simulink model "BallAndPlate_RLSMPC_Controller"  (R2022b)
settings: configuration reference "controller_config_MPC" (kept outside this file)
undefined symbols (not defined in the file): BallAndPlate_ss_d, TimeStep_MPC, V_refNum
libraries: mpclib x1, sharedTrackingLibrary x1
settings Model: DataDictionary=BallAndPlate_system_data.sldd  Creator=tshintai  LastModifiedBy=tshintai
settings ConfigSetRef: SourceName=controller_config_MPC

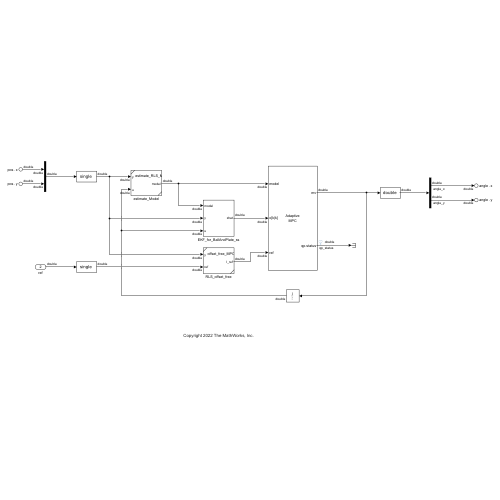
[thumbnail: Simulink's stored preview of the top-level diagram]
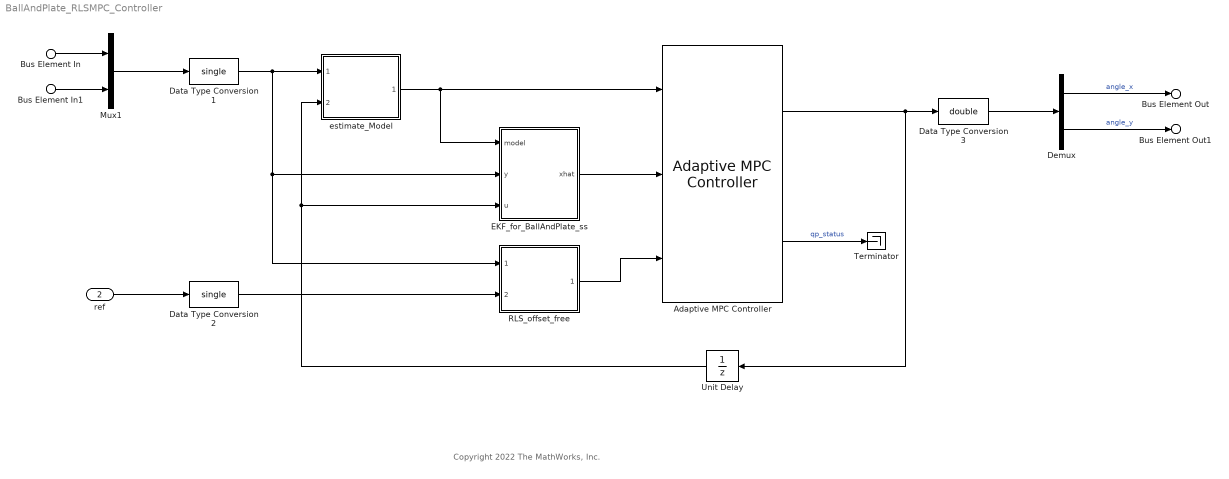
== system BallAndPlate_RLSMPC_Controller ==
  note: Copyright 2022 The MathWorks, Inc.
  Bus Element In : Inport  PortName=pos  Element=x
  Bus Element In1 : Inport  PortName=pos  Element=y
  ref : Inport  Port=2  OutDataTypeStr=double  PortDimensions=[2, V_refNum]
  Adaptive MPC Controller : mpclib/Adaptive MPC Controller  SCDEnableBlockLinearizationSpecification=on  mpcobj=mpcObj_RLS  enable_value=0  updateMPCinCallerWorkspace=on  md_inport=off  mv_inport=off  uref_inport=off  return_cost=off  return_mvseq=off  return_qpstatus=on  return_xseq=off  return_state=off  return_ovseq=off  state_inport=on  isltv_plant=off  umin_inport=off  umax_inport=off  ymin_inport=off  ymax_inport=off  cc_inport=off  ywt_inport=off  uwt_inport=off  duwt_inport=off  rhoeps_inport=off  pm_inport=off  MaximumP=10  HorizonChoice=FixedHorizon  BlockDataType=single  SampleTimeInherited=off  switch_inport=off
  Data Type Conversion1 : DataTypeConversion  OutDataTypeStr=single  SaturateOnIntegerOverflow=off  RndMeth=Floor
  Data Type Conversion2 : DataTypeConversion  OutDataTypeStr=single  SaturateOnIntegerOverflow=off  RndMeth=Floor
  Data Type Conversion3 : DataTypeConversion  OutDataTypeStr=double  SaturateOnIntegerOverflow=off  RndMeth=Floor
  Demux : Demux  Outputs=2
  EKF_for_BallAndPlate_ss : Subsystem
  Mux1 : Mux  Inputs=2
  RLS_offset_free : Subsystem  ReferencedSubsystem=offset_free_MPC
  Terminator : Terminator
  Unit Delay : UnitDelay  SampleTime=-1  HasFrameUpgradeWarning=on
  estimate_Model : Subsystem  ReferencedSubsystem=estimate_RLS_MPC_Model
  Bus Element Out : Outport  PortName=angle  Element=x
  Bus Element Out1 : Outport  PortName=angle  Element=y
  wires:
  Bus Element In/1 -> Mux1/1
  Bus Element In1/1 -> Mux1/2
  Adaptive MPC Controller/2 -> Terminator/1  "qp_status"
  Data Type Conversion2/1 -> RLS_offset_free/2
  estimate_Model/1 -> EKF_for_BallAndPlate_ss/1(model), Adaptive MPC Controller/1
  Adaptive MPC Controller/1 -> Data Type Conversion3/1, Unit Delay/1
  EKF_for_BallAndPlate_ss/1(xhat) -> Adaptive MPC Controller/2
  Unit Delay/1 -> estimate_Model/2, EKF_for_BallAndPlate_ss/3(u)
  Data Type Conversion1/1 -> EKF_for_BallAndPlate_ss/2(y), RLS_offset_free/1, estimate_Model/1
  Data Type Conversion3/1 -> Demux/1
  Mux1/1 -> Data Type Conversion1/1
  ref/1 -> Data Type Conversion2/1
  Demux/1 -> Bus Element Out/1  "angle_x"
  Demux/2 -> Bus Element Out1/1  "angle_y"
  RLS_offset_free/1 -> Adaptive MPC Controller/3

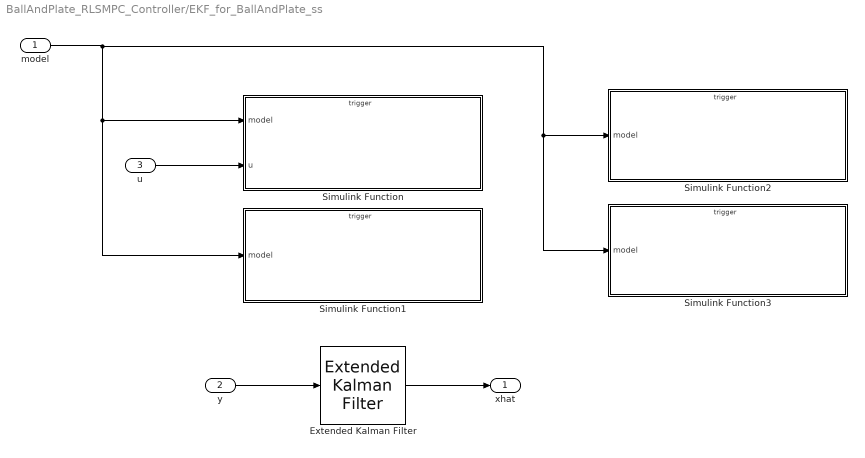
== system BallAndPlate_RLSMPC_Controller/EKF_for_BallAndPlate_ss ==
  model : Inport
  y : Inport  Port=2
  u : Inport  Port=3
  Extended Kalman Filter : sharedTrackingLibrary/Extended Kalman Filter  StateTransitionFcn=EKF_BAP_State_function  HasStateTransitionJacobianFcn=on  StateTransitionJacobianFcn=EKF_BAP_State_Jacobian  HasAdditiveProcessNoise=Additive  ProcessNoise=EKF_Q  HasTimeVaryingProcessNoise=off  HasStateTransitionFcnExtraArgument=0  InitialState=EKF_x_init  InitialStateCovariance=EKF_P_init  MeasurementFcn1=EKF_BAP_Measurement_function  HasMeasurementJacobianFcn1=on  MeasurementJacobianFcn1=EKF_BAP_Measurement_Jacobian  HasMeasurementEnablePort1=off  HasAdditiveMeasurementNoise1=Additive  MeasurementNoise1=EKF_R  HasTimeVaryingMeasurementNoise1=off  HasMeasurementFcnExtraArgument1=0  HasMeasurementWrapping1=off  MeasurementFcn2=myMeasurementFcn  HasMeasurementJacobianFcn2=off  HasMeasurementEnablePort2=off  HasAdditiveMeasurementNoise2=Additive  MeasurementNoise2=1  HasTimeVaryingMeasurementNoise2=off  HasMeasurementFcnExtraArgument2=0  HasMeasurementWrapping2=off  MeasurementFcn3=myMeasurementFcn  HasMeasurementJacobianFcn3=off  HasMeasurementEnablePort3=off  HasAdditiveMeasurementNoise3=Additive  MeasurementNoise3=1  HasTimeVaryingMeasurementNoise3=off  HasMeasurementFcnExtraArgument3=0  HasMeasurementWrapping3=off  MeasurementFcn4=myMeasurementFcn  HasMeasurementJacobianFcn4=off  HasMeasurementEnablePort4=off  HasAdditiveMeasurementNoise4=Additive  MeasurementNoise4=1  HasTimeVaryingMeasurementNoise4=off  HasMeasurementFcnExtraArgument4=0  HasMeasurementWrapping4=off  MeasurementFcn5=myMeasurementFcn  HasMeasurementJacobianFcn5=off  HasMeasurementEnablePort5=off  HasAdditiveMeasurementNoise5=Additive  MeasurementNoise5=1  HasTimeVaryingMeasurementNoise5=off  HasMeasurementFcnExtraArgument5=0  HasMeasurementWrapping5=off  EnableMultirate=off  StateTransitionFcnSampleTime=1  MeasurementFcn1SampleTime=1  MeasurementFcn2SampleTime=1  MeasurementFcn3SampleTime=1  MeasurementFcn4SampleTime=1  MeasurementFcn5SampleTime=1  UseCurrentEstimator=on  OutputStateCovariance=off  DataType=single  SampleTime=TimeStep_MPC  NumberOfMeasurements=1
  Simulink Function : Subsystem  TreatAsAtomicUnit=on
  Simulink Function1 : Subsystem  TreatAsAtomicUnit=on
  Simulink Function2 : Subsystem  TreatAsAtomicUnit=on
  Simulink Function3 : Subsystem  TreatAsAtomicUnit=on
  xhat : Outport
  wires:
  u/1 -> Simulink Function/2(u)
  Extended Kalman Filter/1 -> xhat/1
  y/1 -> Extended Kalman Filter/1
  model/1 -> Simulink Function1/1(model), Simulink Function/1(model), Simulink Function3/1(model), Simulink Function2/1(model)

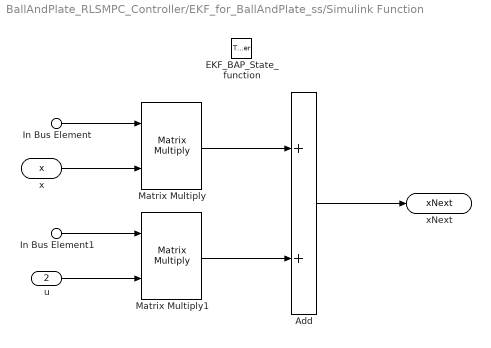
== system BallAndPlate_RLSMPC_Controller/EKF_for_BallAndPlate_ss/Simulink Function ==
  In Bus Element : Inport  PortName=model  Element=A
  In Bus Element1 : Inport  PortName=model  Element=B
  u : Inport  Port=2
  EKF_BAP_State_function : TriggerPort  TriggerType=function-call  IsSimulinkFunction=on  FunctionName=EKF_BAP_State_function  FunctionVisibility=scoped  VariantControl=(inherit)
  Add : Sum
  Matrix Multiply : Product  Multiplication=Matrix(*)
  Matrix Multiply1 : Product  Multiplication=Matrix(*)
  x : ArgIn  DisableCoverage=on  OutDataTypeStr=single  PortDimensions=size(BallAndPlate_ss_d.A, 1)  ArgumentName=x
  xNext : ArgOut  DisableCoverage=on  OutDataTypeStr=single  PortDimensions=size(BallAndPlate_ss_d.A, 1)  ArgumentName=xNext
  wires:
  x/1 -> Matrix Multiply/2
  In Bus Element/1 -> Matrix Multiply/1
  u/1 -> Matrix Multiply1/2
  In Bus Element1/1 -> Matrix Multiply1/1
  Matrix Multiply/1 -> Add/1
  Matrix Multiply1/1 -> Add/2
  Add/1 -> xNext/1

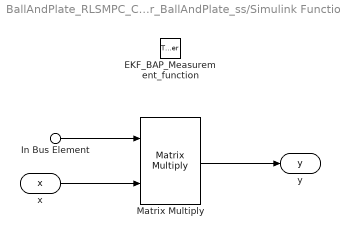
== system BallAndPlate_RLSMPC_Controller/EKF_for_BallAndPlate_ss/Simulink Function1 ==
  In Bus Element : Inport  PortName=model  Element=C
  EKF_BAP_Measurement_function : TriggerPort  TriggerType=function-call  IsSimulinkFunction=on  FunctionName=EKF_BAP_Measurement_function  FunctionVisibility=scoped  VariantControl=(inherit)
  Matrix Multiply : Product  Multiplication=Matrix(*)
  x : ArgIn  DisableCoverage=on  OutDataTypeStr=single  PortDimensions=size(BallAndPlate_ss_d.A, 1)  ArgumentName=x
  y : ArgOut  DisableCoverage=on  OutDataTypeStr=single  PortDimensions=size(BallAndPlate_ss_d.C, 1)  ArgumentName=y
  wires:
  In Bus Element/1 -> Matrix Multiply/1
  x/1 -> Matrix Multiply/2
  Matrix Multiply/1 -> y/1

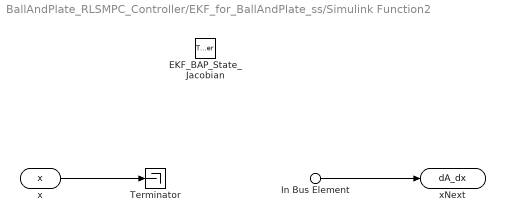
== system BallAndPlate_RLSMPC_Controller/EKF_for_BallAndPlate_ss/Simulink Function2 ==
  In Bus Element : Inport  PortName=model  Element=A
  EKF_BAP_State_Jacobian : TriggerPort  TriggerType=function-call  IsSimulinkFunction=on  FunctionName=EKF_BAP_State_Jacobian  FunctionVisibility=scoped  VariantControl=(inherit)
  Terminator : Terminator
  x : ArgIn  DisableCoverage=on  OutDataTypeStr=single  PortDimensions=size(BallAndPlate_ss_d.A, 1)  ArgumentName=x
  xNext : ArgOut  DisableCoverage=on  OutDataTypeStr=single  PortDimensions=size(BallAndPlate_ss_d.A)  ArgumentName=dA_dx
  wires:
  In Bus Element/1 -> xNext/1
  x/1 -> Terminator/1

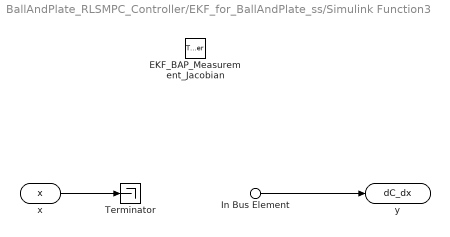
== system BallAndPlate_RLSMPC_Controller/EKF_for_BallAndPlate_ss/Simulink Function3 ==
  In Bus Element : Inport  PortName=model  Element=C
  EKF_BAP_Measurement_Jacobian : TriggerPort  TriggerType=function-call  IsSimulinkFunction=on  FunctionName=EKF_BAP_Measurement_Jacobian  FunctionVisibility=scoped  VariantControl=(inherit)
  Terminator : Terminator
  x : ArgIn  DisableCoverage=on  OutDataTypeStr=single  PortDimensions=size(BallAndPlate_ss_d.A, 1)  ArgumentName=x
  y : ArgOut  DisableCoverage=on  OutDataTypeStr=single  PortDimensions=size(BallAndPlate_ss_d.C)  ArgumentName=dC_dx
  wires:
  In Bus Element/1 -> y/1
  x/1 -> Terminator/1
